simulink subsystem "WSS"  (R2025b)
settings: Solver=VariableStepAuto  StartTime=0.0  StopTime=10.0  RelTol=1e-3
libraries: hdlsllib x2
settings Model: Creator=diego  LastModifiedBy=diego

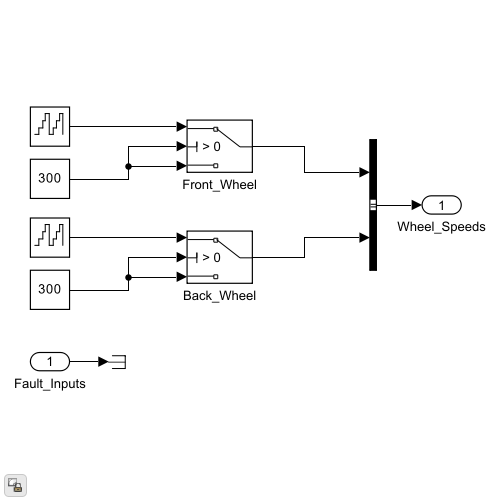
[thumbnail: Simulink's stored preview of the top-level diagram]
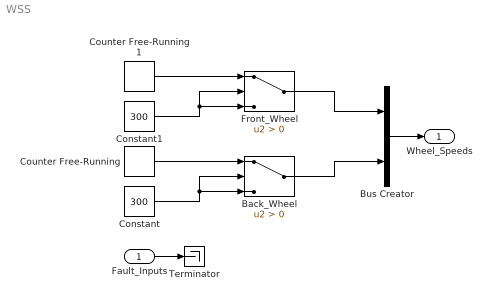
== system WSS ==
  Fault_Inputs : Inport
  Back_Wheel : Switch  Criteria=u2 > Threshold  SaturateOnIntegerOverflow=off  InputSameDT=off
  Bus Creator : BusCreator  Inputs=2
  Constant : Constant  Value=300
  Constant1 : Constant  Value=300
  Counter Free-Running : hdlsllib/Sources/Counter Free-Running  NumBits=16  tsamp=-1
  Counter Free-Running1 : hdlsllib/Sources/Counter Free-Running  NumBits=16  tsamp=-1
  Front_Wheel : Switch  Criteria=u2 > Threshold  SaturateOnIntegerOverflow=off  InputSameDT=off
  Terminator : Terminator
  Wheel_Speeds : Outport
  wires:
  Back_Wheel/1 -> Bus Creator/2
  Counter Free-Running/1 -> Back_Wheel/1
  Constant/1 -> Back_Wheel/3, Back_Wheel/2
  Fault_Inputs/1 -> Terminator/1
  Front_Wheel/1 -> Bus Creator/1
  Counter Free-Running1/1 -> Front_Wheel/1
  Constant1/1 -> Front_Wheel/3, Front_Wheel/2
  Bus Creator/1 -> Wheel_Speeds/1
